simulink model "ControlTask1"  (R2023b)
settings: Solver=VariableStepAuto  StartTime=0.0  StopTime=100  RelTol=1e-3
libraries: slpidlib x1
settings Model: Creator=Ashutosh Joshi  LastModifiedBy=Ashutosh Joshi

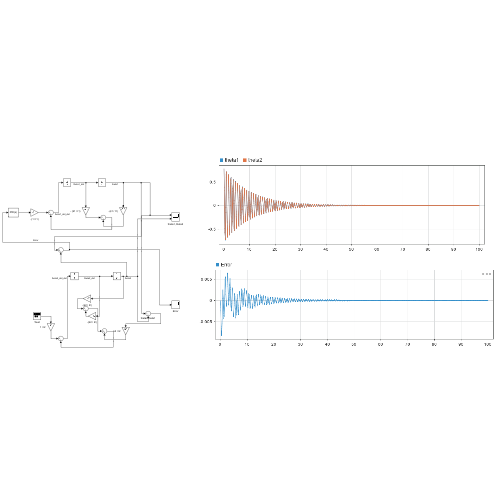
[thumbnail: Simulink's stored preview of the top-level diagram]
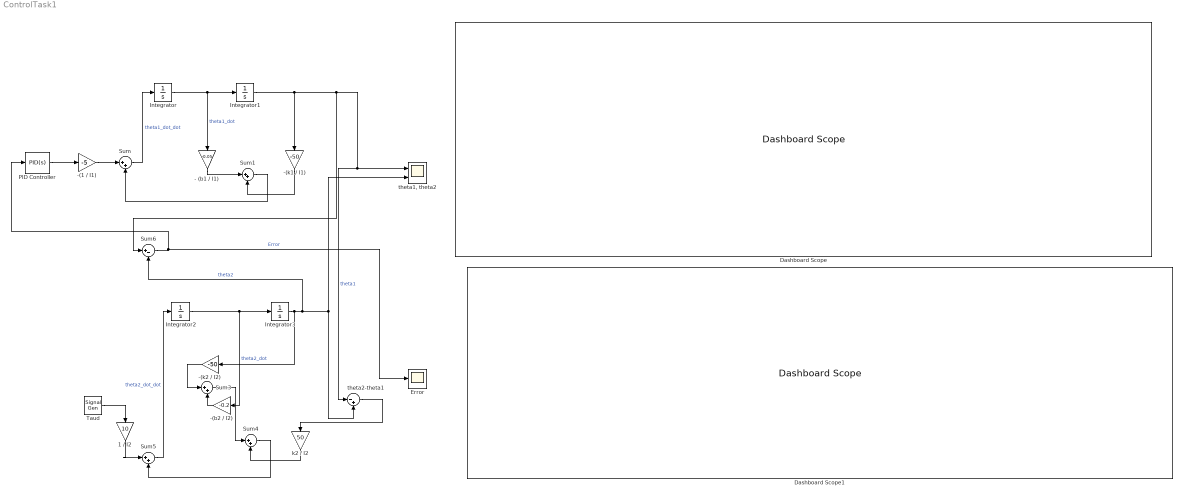
== system ControlTask1 ==
  - (b1 / I1) : Gain  Gain=-0.05
  -(1 / I1) : Gain  Gain=-5
  -(b2 / I2) : Gain  Gain=-0.2
  -(k1 / I1) : Gain  Gain=-50
  -(k2 / I2) : Gain  Gain=-50
  1 / I2 : Gain  Gain=10
  Dashboard Scope : DashboardScope  NormalizeYAxis=on
  Dashboard Scope1 : DashboardScope
  Error : Scope
  Integrator : Integrator
  Integrator1 : Integrator  InitialCondition=pi/4
  Integrator2 : Integrator
  Integrator3 : Integrator  InitialCondition=pi/4
  PID Controller : slpidlib/PID Controller  Controller=PID  Form=Parallel  TimeDomain=Continuous-time  UseExternalTs=off  SampleTime=-1  IntegratorMethod=Forward Euler  FilterMethod=Forward Euler  ControllerParametersSource=internal  P=2.4  I=5.5122  UseKiTs=off  D=5  N=100  UseFilter=on  TunerSelectOption=Transfer Function Based (PID Tuner App)  InitialConditionSource=internal  InitialConditionForIntegrator=0  InitialConditionForFilter=0  DifferentiatorICPrevScaledInput=0  ExternalReset=none  TrackingMode=off  Kt=1  LimitOutput=off  SatLimitsSource=internal  UpperSaturationLimit=inf  LowerSaturationLimit=-inf  LinearizeAsGain=on  AntiWindupMode=none  Kb=1  LimitIntegrator=off  UpperIntegratorSaturationLimit=inf  LowerIntegratorSaturationLimit=-inf  POutMin=[]  POutMax=[]  IOutMin=[]  IOutMax=[]  DOutMin=[]  DOutMax=[]  NOutMin=[]  NOutMax=[]  SumOutMin=[]  SumOutMax=[]  SaturationOutMin=[]  SaturationOutMax=[]  PParamMin=[]  PParamMax=[]  IParamMin=[]  IParamMax=[]  DParamMin=[]  DParamMax=[]  NParamMin=[]  NParamMax=[]  KbParamMin=[]  KbParamMax=[]  KtParamMin=[]  KtParamMax=[]  KbOutMin=[]  KbOutMax=[]  KtOutMin=[]  KtOutMax=[]  IntegratorOutMin=[]  IntegratorOutMax=[]  FilterOutMin=[]  FilterOutMax=[]  SumI1OutMin=[]  SumI1OutMax=[]  SumI2OutMin=[]  SumI2OutMax=[]  SumI3OutMin=[]  SumI3OutMax=[]  SumI4OutMin=[]  SumI4OutMax=[]  SumDOutMin=[]  SumDOutMax=[]  DifferentiatorOutMin=[]  DifferentiatorOutMax=[]  FilterDiffOutCoefMin=[]  FilterDiffOutCoefMax=[]  ReciprocalOutMin=[]  ReciprocalOutMax=[]  SumDenOutMin=[]  SumDenOutMax=[]  SumNumOutMin=[]  SumNumOutMax=[]  DivideOutMin=[]  DivideOutMax=[]  UdiffTsProdOutMin=[]  UdiffTsProdOutMax=[]  NTsProdOutMin=[]  NTsProdOutMax=[]  UintegralTsProdOutMin=[]  UintegralTsProdOutMax=[]  UngainTsProdOutMin=[]  UngainTsProdOutMax=[]  ClampingZeroOutDataTypeStr=Inherit: Inherit via back propagation  ClampingZeroOutMin=[]  ClampingZeroOutMax=[]  FilterDenConstantOutDataTypeStr=Inherit: Inherit via back propagation  FilterDenConstantOutMin=[]  FilterDenConstantOutMax=[]  PCopyOutDataTypeStr=Inherit: Inherit via back propagation  PCopyOutMin=[]  PCopyOutMax=[]  NCopyOutDataTypeStr=Inherit: Inherit via back propagation  NCopyOutMin=[]  NCopyOutMax=[]  IntegratorContinuousStateAttributes=''  IntegratorStateMustResolveToSignalObject=off  IntegratorRTWStateStorageClass=Auto  FilterContinuousStateAttributes=''  FilterStateMustResolveToSignalObject=off  FilterRTWStateStorageClass=Auto  ParallelPVariant=InternalParameters  IdealPVariant=Disabled  IVariant=InternalParameters  DVariant=InternalParameters  IntegratorVariant=Continuous  SatVariant=Disabled  AWVariant=Passthrough  PCopyVariant=Disabled  TRVariant=Disabled  FdbkBlocksVariant=Forward  IdealPFdbkVariant=Disabled  SatFdbkVariant=Disabled  DerivativeFilterVariant=ContFilter  NVariant=InternalParameters  NCopyVariant=Disabled  FilterICVariant=InternalICsFilter  IntegratorICVariant=InternalICs  ExternalResetVariant=Disabled  TRSumVariant=Passthrough  SumFdbkVariant=Disabled  SumVariant=Sum_PID  TsampFilterVariant=InternalTs  TsampNgainVariant=Passthrough  TsampIntegralVariant=Disabled_SignalSpec  ExternalSaturationOutDataTypeStr=Inherit: Same as second input
  Sum{,1,3..5} (5 alike) : Sum  Inputs=|++
  Sum6 : Sum  Inputs=|+-
  Taud : SignalGenerator  Amplitude=0.05  Frequency=100  Units=rad/sec
  k2 / I2 : Gain  Gain=50
  "theta1, theta2" : Scope  NumInputPorts=2
  theta2-theta1 : Sum  Inputs=|-+
  wires:
  Integrator/1 -> - (b1 / I1)/1, Integrator1/1  "theta1_dot"
  Integrator1/1 -> Sum6/1, theta2-theta1/1, "theta1, theta2"/1, -(k1 / I1)/1  "theta1"
  Sum/1 -> Integrator/1  "theta1_dot_dot"
  -(k1 / I1)/1 -> Sum1/2
  - (b1 / I1)/1 -> Sum1/1
  Sum1/1 -> Sum/2
  PID Controller/1 -> -(1 / I1)/1
  -(1 / I1)/1 -> Sum/1
  Integrator2/1 -> Integrator3/1, -(b2 / I2)/1  "theta2_dot"
  Sum5/1 -> Integrator2/1  "theta2_dot_dot"
  Integrator3/1 -> -(k2 / I2)/1, theta2-theta1/2, "theta1, theta2"/2, Sum6/2  "theta2"
  -(b2 / I2)/1 -> Sum3/2
  -(k2 / I2)/1 -> Sum3/1
  Sum3/1 -> Sum4/1
  theta2-theta1/1 -> k2 / I2/1
  k2 / I2/1 -> Sum4/2
  Sum4/1 -> Sum5/2
  Taud/1 -> 1 / I2/1
  1 / I2/1 -> Sum5/1
  Sum6/1 -> PID Controller/1, Error/1  "Error"
